simulink model "Zad2"  (R2020b)
settings: Solver=VariableStepAuto  StartTime=0.0  StopTime=0.0  RelTol=1e-3
libraries: CPOiS_SourcesSinks x11, CPOiS_Filters x6, CPOiS_DataManipulation_IntroduceNoise x2, CPOiS_DataManipulation_DataTypeConversion x2, CPOiS_General x1
settings Model: Creator=Krystian  LastModifiedBy=Krystian

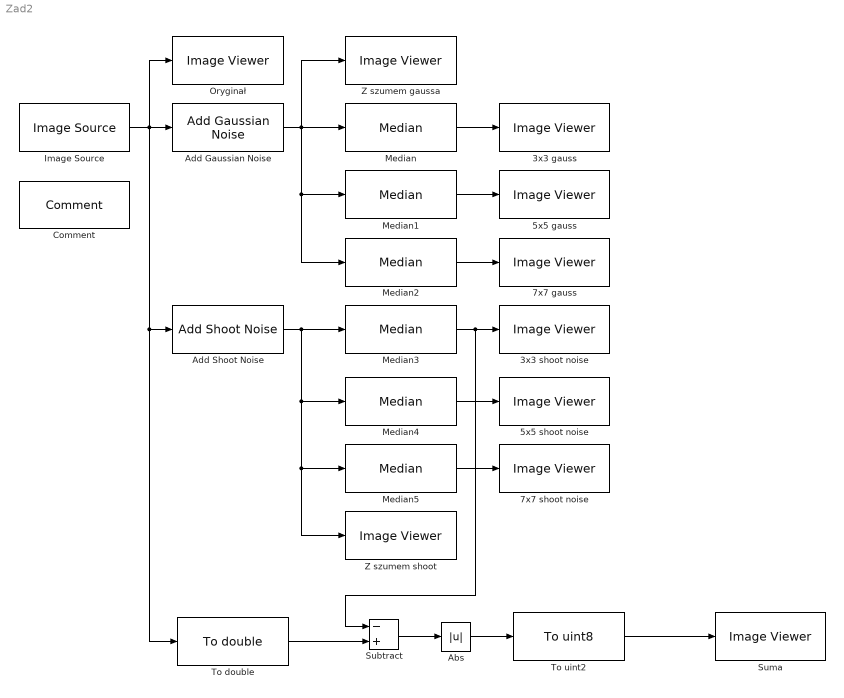
== system Zad2 ==
  3x3 gauss : CPOiS_SourcesSinks/Image Viewer
      settings: SourceProductName=CPOiS - Digital image and signal processing
  "3x3 shoot noise " : CPOiS_SourcesSinks/Image Viewer
      settings: SourceProductName=CPOiS - Digital image and signal processing
  5x5 gauss : CPOiS_SourcesSinks/Image Viewer
      settings: SourceProductName=CPOiS - Digital image and signal processing
  "5x5 shoot noise " : CPOiS_SourcesSinks/Image Viewer
      settings: SourceProductName=CPOiS - Digital image and signal processing
  7x7 gauss : CPOiS_SourcesSinks/Image Viewer
      settings: SourceProductName=CPOiS - Digital image and signal processing
  7x7 shoot noise : CPOiS_SourcesSinks/Image Viewer
      settings: SourceProductName=CPOiS - Digital image and signal processing
  Abs : Abs
  Add Gaussian Noise : CPOiS_DataManipulation_IntroduceNoise/Add Gaussian Noise  Mean=0  Variance=1
      settings: SourceProductName=CPOiS - Digital image and signal processing
  Add Shoot Noise : CPOiS_DataManipulation_IntroduceNoise/Add Shoot Noise  Density=5
      settings: SourceProductName=CPOiS - Digital image and signal processing
  Comment : CPOiS_General/Comment
      settings: SourceProductName=CPOiS - Digital image and signal processing
  Image Source : CPOiS_SourcesSinks/Image Source  FileSelection=ball.png
      settings: SourceProductName=CPOiS - Digital image and signal processing
  Median{,1..5} (6 alike) : CPOiS_Filters/Median
      settings: SourceProductName=CPOiS - Digital image and signal processing
  Oryginał : CPOiS_SourcesSinks/Image Viewer
      settings: SourceProductName=CPOiS - Digital image and signal processing
  Subtract : Sum  Inputs=-+
  Suma : CPOiS_SourcesSinks/Image Viewer
      settings: SourceProductName=CPOiS - Digital image and signal processing
  To double : CPOiS_DataManipulation_DataTypeConversion/To double
      settings: SourceProductName=CPOiS - Digital image and signal processing
  To uint2 : CPOiS_DataManipulation_DataTypeConversion/To uint8
      settings: SourceProductName=CPOiS - Digital image and signal processing
  "Z szumem gaussa " : CPOiS_SourcesSinks/Image Viewer
      settings: SourceProductName=CPOiS - Digital image and signal processing
  Z szumem shoot : CPOiS_SourcesSinks/Image Viewer
      settings: SourceProductName=CPOiS - Digital image and signal processing
  wires:
  Add Shoot Noise/1 -> Z szumem shoot/1, Median5/1, Median4/1, Median3/1
  Median/1 -> 3x3 gauss/1
  Median5/1 -> 7x7 shoot noise/1
  Median4/1 -> "5x5 shoot noise "/1
  Median2/1 -> 7x7 gauss/1
  Add Gaussian Noise/1 -> Median1/1, Median2/1, Median/1, "Z szumem gaussa "/1
  Median1/1 -> 5x5 gauss/1
  Image Source/1 -> Add Gaussian Noise/1, To double/1, Add Shoot Noise/1, Oryginał/1
  Abs/1 -> To uint2/1
  To double/1 -> Subtract/2
  Subtract/1 -> Abs/1
  To uint2/1 -> Suma/1
  Median3/1 -> "3x3 shoot noise "/1, Subtract/1
